simulink model "march24example1"  (R2023b)
settings: Solver=VariableStepAuto  StartTime=0.0  StopTime=3600  RelTol=1e-3
undefined symbols (not defined in the file): Ion, Lithium
libraries: spsBatteryLib x1, spsControlledCurrentSourceLib x1, sps_lib x1
settings Model: Creator=ray  LastModifiedBy=ray

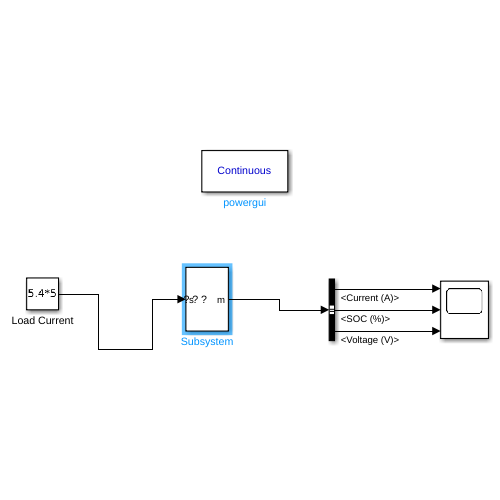
[thumbnail: Simulink's stored preview of the top-level diagram]
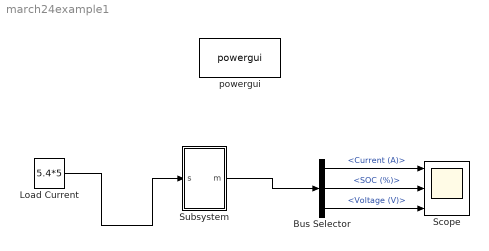
== system march24example1 ==
  Bus Selector : BusSelector  OutputSignals=Current (A),SOC (%),Voltage (V)
  Load Current : Constant  Value=5.4*5
  Scope : Scope  NumInputPorts=3
  Subsystem : Subsystem
      mask Display: image('battery-charging-concept-glowing-icon-charged-battery-d-render_120871-816.webp');
  powergui : sps_lib/powergui  Priority=1  SimulationMode=Continuous  SampleTime=50e-6  frequency=60  Iterations=50  frequencyindice=0  Pbase=100e6  ErrMax=1e-4  UnitsV=kV  UnitsW=MW  buscounter=0  FunctionMessages=off  echomessages=off  EnableUseOfTLC=off  CurrentSourceSwitches=off  DisableSnubberDevices=off  DisableRonSwitches=off  DisableVfSwitches=off  DisplayEquations=off  AutomaticDiscreteSolvers=off  SolverType=Tustin/Backward Euler (TBE)  Interpol=off  ExternalGateDelay=off  methode=off  Ts=100  x0status=blocks  SPID=on  SwTol=0  HookPort=off  NonlinearTolerance=1e-4  nMaxIteration=100  ContinueOnMaxIteration=off  RestoreLinks=warning  ResistiveCurrentMeasurement=off  Frange=[0:2:500]  Ylog=off  Xlog=on  ShowGrid=off  save=off  variable=ZData  structure=0  ZoomFFT=off  StartTime=0.0  cycles=1  DisplayStyle=1  fundamental=60  FreqAxis=off  MaxFrequency=1000  frequencyindicesteady=1  RmsSteady=1  display=off
  wires:
  Bus Selector/1 -> Scope/1  "<Current (A)>"
  Bus Selector/2 -> Scope/2  "<SOC (%)>"
  Bus Selector/3 -> Scope/3  "<Voltage (V)>"
  Load Current/1 -> Subsystem/1(s)
  Subsystem/1(m) -> Bus Selector/1

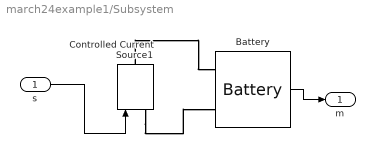
== system march24example1/Subsystem ==
  s : Inport
  Battery : spsBatteryLib/Battery  BatType=Lithium-Ion  ShowTempParam=off  ThermalPreset=no  ShowAgeParam=off  NomV=7.2  NomQ=54  SOC=100  Batt_Tr=30  PresetModel=on  MaxQ=54  MinV=5.4  FullV=8.3807  Dis_rate=23.4783  R=0.0013333  Normal_OP=48.8348  expZone="[7.7788       2.653]"  current=[6.5 13 32.5]  Units=Time  Tci=20  NomT=20  T2=-30  MaxQ2=4.8  FullV2=7.1  Normal_OP2=5.655  expZone2="[6.58           1]"  Rca=0.6  ti=2000  Dp=0  Neq0=0  Tsim=1e6  Ta1=25  Qeol=5.4*0.9  Reol=0.013333*1.2  Char_age=[2.3478, 3]  Dis_age=[2.3478, 10]  N1=1500  N2=10500  N3=1000  N4=1400  Ta2=45  N5=950
  Controlled Current Source1 : spsControlledCurrentSourceLib/Controlled Current Source  Initialize=on  Source_Type=AC  Amplitude=0  Phase=0  Frequency=0  Measurements=None
  m : Outport
  wires:
  s/1 -> Controlled Current Source1/1
  Battery/1 -> m/1
  connections:
  Controlled Current Source1/LConn1 -- Battery/LConn1
  Controlled Current Source1/RConn1 -- Battery/LConn2
